simulink model "FOZN_BlueROV2_Control"  (R2023b)
settings: Solver=FixedStepAuto  StartTime=0.0  StopTime=600  FixedStep=0.01  RelTol=1e-3
values from neighbouring files (symbols this model uses):
  app_order = 5    [FOZN_controllers.m]
  Kp_heave = 0.2*Kc    (= 0.905736827128)    [RelayTest_controllerCalc.m]
  Kp_pitch = 0.2*Kc    (= 1.14706265291)    [RelayTest_controllerCalc.m]
  Kp_roll = 0.2*Kc    (= 0.102773850851)    [RelayTest_controllerCalc.m]
  Kp_surge = 0.2*Kc    (= 1.80686784967)    [RelayTest_controllerCalc.m]
  Kp_sway = 0.2*Kc    (= 0.383313460532)    [RelayTest_controllerCalc.m]
  Kp_yaw = 0.2*Kc    (= 0.127394021185)    [RelayTest_controllerCalc.m]
undefined symbols (not defined in the file or in its folder): Td_heave, Td_pitch, Td_roll, Td_surge, Td_sway, Td_yaw, Ti_heave, Ti_pitch, Ti_roll, Ti_surge, Ti_sway, Ti_yaw
libraries: fod x12
settings Model: Creator=tudor  LastModifiedBy=tudor

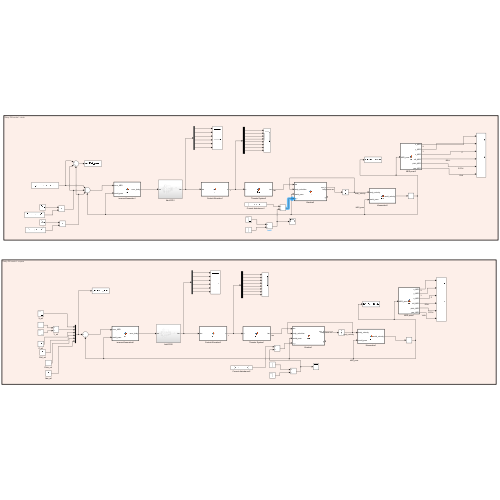
[thumbnail: Simulink's stored preview of the top-level diagram]
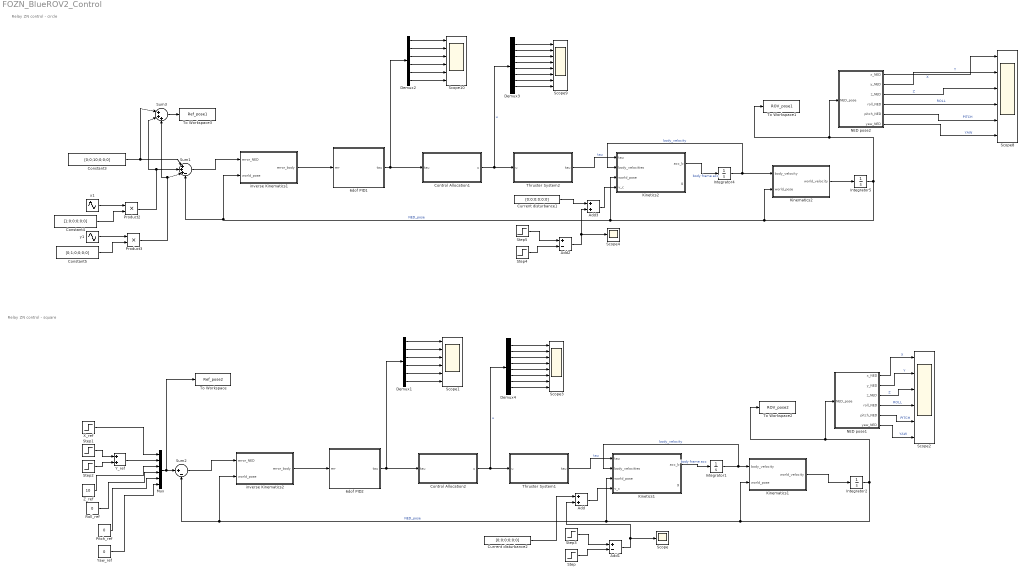
== system FOZN_BlueROV2_Control ==
  note: Relay ZN control - circle
  note: Relay ZN control - square
  6dof PID1 : Subsystem
  6dof PID2 : Subsystem
  Add : Sum
  Add1 : Sum  Inputs=+-
  Add2 : Sum  Inputs=+-
  Add3 : Sum
  Constant3 : Constant  Value=[0;0;10;0;0;0]
  Constant4 : Constant  Value=[1;0;0;0;0;0]
  Constant5 : Constant  Value=[0;1;0;0;0;0]
  Control Allocation1 : MATLAB Function  TreatAsAtomicUnit=on
  Control Allocation2 : MATLAB Function  TreatAsAtomicUnit=on
  Current disturbance1 : Constant  Value=[0;0;0;0;0;0]
  Current disturbance2 : Constant  Value=[0;0;0;0;0;0]
  Demux1 : Demux  Outputs=6
  Demux2 : Demux  Outputs=6
  Demux3 : Demux  Outputs=8
  Demux4 : Demux  Outputs=8
  Integrator1 : Integrator  InitialCondition=[0;0;0;0;0;0]
  Integrator2 : Integrator  InitialCondition=[0;0;10;0;0;0]
  Integrator4 : Integrator  InitialCondition=[0;0;0;0;0;0]
  Integrator5 : Integrator  InitialCondition=[0;0;10;0;0;0]
  Kinematics1 : MATLAB Function  TreatAsAtomicUnit=on
  Kinematics2 : MATLAB Function  TreatAsAtomicUnit=on
  Kinetics1 : MATLAB Function  TreatAsAtomicUnit=on
  Kinetics2 : MATLAB Function  TreatAsAtomicUnit=on
  Mux : Mux  Inputs=6
  NED pose1 : MATLAB Function  TreatAsAtomicUnit=on
  NED pose2 : MATLAB Function  TreatAsAtomicUnit=on
  Pitch_ref : Constant  Value=0
  Product2 : Product
  Product3 : Product
  Roll_ref : Constant  Value=0
  Scope : Scope
  Scope{1..2,8,10} (4 alike) : Scope  NumInputPorts=6
  Scope3 : Scope  NumInputPorts=8
  Scope4 : Scope
  Scope9 : Scope  NumInputPorts=8
  Step : Step  Time=100  Before=0.45  After=0  SampleTime=0
  Step1 : Step  Time=150  After=5  SampleTime=0
  Step2 : Step  Time=450  After=-5  SampleTime=0
  Step3 : Step  Time=125  Before=0.45  After=0  SampleTime=0
  Step4 : Step  Time=100  Before=0.45  After=0  SampleTime=0
  Step5 : Step  Time=125  Before=0.45  After=0  SampleTime=0
  Sum1 : Sum  Inputs=|+++-
  Sum2 : Sum  Inputs=|+-
  Sum3 : Sum  Inputs=|+++
  Thruster System1 : MATLAB Function  TreatAsAtomicUnit=on
  Thruster System2 : MATLAB Function  TreatAsAtomicUnit=on
  To Workspace : ToWorkspace  VariableName=Ref_pose2  SampleTime=-1
  To Workspace1 : ToWorkspace  VariableName=ROV_pose1  SampleTime=-1
  To Workspace2 : ToWorkspace  VariableName=ROV_pose2  SampleTime=-1
  To Workspace3 : ToWorkspace  VariableName=Ref_pose1  SampleTime=-1
  X_ref : Step  Time=300  Before=5  After=0  SampleTime=0
  Y_ref : Sum
  Yaw_ref : Constant  Value=0
  Z_ref : Constant  Value=10
  inverse Kinematics1 : MATLAB Function  TreatAsAtomicUnit=on
  inverse Kinematics2 : MATLAB Function  TreatAsAtomicUnit=on
  x1 : Sin  Frequency=0.1  SampleTime=0
  y1 : Sin  Frequency=0.1  Phase=pi/2  SampleTime=0
  wires:
  Demux2/6 -> Scope10/6
  Kinematics2/1(world_velocity) -> Integrator5/1
  Control Allocation1/1(u) -> Demux3/1, Thruster System2/1(u)  "u"
  NED pose2/6(yaw_NED) -> Scope8/6  "YAW"
  Demux3/3 -> Scope9/3
  Demux3/6 -> Scope9/6
  Demux3/2 -> Scope9/2
  Demux2/1 -> Scope10/1
  Kinetics2/1(acc_b) -> Integrator4/1  "body frame acc"
  Demux2/3 -> Scope10/3
  inverse Kinematics1/1(error_body) -> 6dof PID1/1(err)
  NED pose2/1(x_NED) -> Scope8/1  "X"
  Demux3/1 -> Scope9/1
  Current disturbance1/1 -> Add3/1
  Sum1/1 -> inverse Kinematics1/1(error_NED)
  Demux3/8 -> Scope9/8
  Integrator4/1 -> Kinetics2/2(body_velocities), Kinematics2/1(body_velocity)  "body_velocity"
  Demux3/7 -> Scope9/7
  Constant3/1 -> Sum3/1, Sum1/1
  6dof PID1/1(tau) -> Demux2/1, Control Allocation1/1(tau)
  Demux2/4 -> Scope10/4
  Thruster System2/1(tau) -> Kinetics2/1(tau)  "tau"
  Demux3/4 -> Scope9/4
  Integrator5/1 -> To Workspace1/1, NED pose2/1(NED_pose), Kinetics2/3(world_pose), Sum1/4, inverse Kinematics1/2(world_pose), Kinematics2/2(world_pose)  "NED_pose"
  NED pose2/2(y_NED) -> Scope8/2  "Y"
  NED pose2/4(roll_NED) -> Scope8/4  "ROLL"
  Demux2/2 -> Scope10/2
  NED pose2/3(z_NED) -> Scope8/3  "Z"
  Demux3/5 -> Scope9/5
  NED pose2/5(pitch_NED) -> Scope8/5  "PITCH"
  Demux2/5 -> Scope10/5
  Constant5/1 -> Product3/2
  Constant4/1 -> Product2/2
  y1/1 -> Product3/1
  Product2/1 -> Sum3/2, Sum1/2
  x1/1 -> Product2/1
  Product3/1 -> Sum1/3, Sum3/3
  X_ref/1 -> Mux/1
  Pitch_ref/1 -> Mux/5
  Step1/1 -> Y_ref/1
  Mux/1 -> To Workspace/1, Sum2/1
  Step2/1 -> Y_ref/2
  Y_ref/1 -> Mux/2
  Z_ref/1 -> Mux/3
  Yaw_ref/1 -> Mux/6
  Roll_ref/1 -> Mux/4
  6dof PID2/1(tau) -> Demux1/1, Control Allocation2/1(tau)
  Demux1/4 -> Scope1/4
  Demux4/8 -> Scope3/8
  Demux1/6 -> Scope1/6
  Control Allocation2/1(u) -> Demux4/1, Thruster System1/1(u)  "u"
  Kinematics1/1(world_velocity) -> Integrator2/1
  NED pose1/6(yaw_NED) -> Scope2/6  "YAW"
  Sum2/1 -> inverse Kinematics2/1(error_NED)
  Demux4/1 -> Scope3/1
  Demux1/1 -> Scope1/1
  Demux1/5 -> Scope1/5
  Kinetics1/1(acc_b) -> Integrator1/1  "body frame acc"
  NED pose1/4(roll_NED) -> Scope2/4  "ROLL"
  Thruster System1/1(tau) -> Kinetics1/1(tau)  "tau"
  Demux4/7 -> Scope3/7
  Demux1/3 -> Scope1/3
  Integrator2/1 -> To Workspace2/1, NED pose1/1(NED_pose), Kinetics1/3(world_pose), Sum2/2, inverse Kinematics2/2(world_pose), Kinematics1/2(world_pose)  "NED_pose"
  NED pose1/1(x_NED) -> Scope2/1  "X"
  inverse Kinematics2/1(error_body) -> 6dof PID2/1(err)
  Demux4/4 -> Scope3/4
  Demux4/6 -> Scope3/6
  Current disturbance2/1 -> Add/1
  NED pose1/5(pitch_NED) -> Scope2/5  "PITCH"
  Demux4/3 -> Scope3/3
  NED pose1/2(y_NED) -> Scope2/2  "Y"
  Demux4/2 -> Scope3/2
  Demux1/2 -> Scope1/2
  Integrator1/1 -> Kinetics1/2(body_velocities), Kinematics1/1(body_velocity)  "body_velocity"
  Demux4/5 -> Scope3/5
  NED pose1/3(z_NED) -> Scope2/3  "Z"
  Add/1 -> Kinetics1/4(v_c)
  Step3/1 -> Add1/1
  Step/1 -> Add1/2
  Add1/1 -> Scope/1, Add/2
  Sum3/1 -> To Workspace3/1
  Add2/1 -> Add3/2, Scope4/1
  Step4/1 -> Add2/2
  Step5/1 -> Add2/1
  Add3/1 -> Kinetics2/4(v_c)

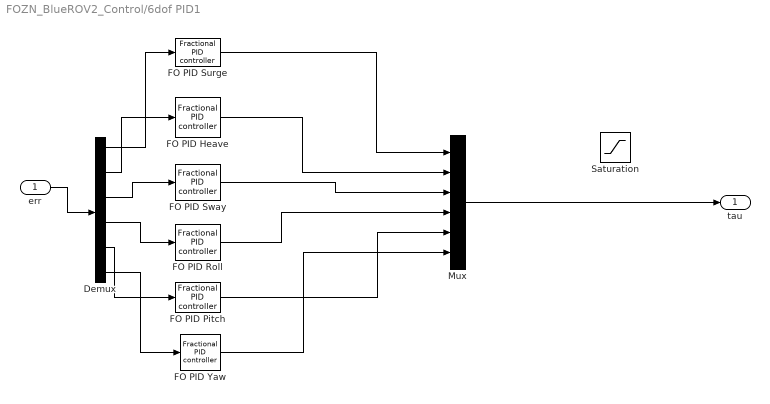
== system FOZN_BlueROV2_Control/6dof PID1 ==
  err : Inport
  Demux : Demux  Outputs=6
  FO PID Heave : fod/Fractional PID controller  Kp=Kp_heave  Ki=Kp_heave/Ti_heave  lambda=lambda_heave  Kd=Kp_heave*Td_heave  mic=lambda_heave  freqRange=freq_range  N=app_order
      settings: SourceProductName=FOMCON Toolbox
  FO PID Pitch : fod/Fractional PID controller  Kp=Kp_pitch  Ki=Kp_pitch/Ti_pitch  lambda=lambda_pitch  Kd=Kp_pitch*Td_pitch  mic=lambda_pitch  freqRange=freq_range  N=app_order
      settings: SourceProductName=FOMCON Toolbox
  FO PID Roll : fod/Fractional PID controller  Kp=Kp_roll  Ki=Kp_roll/Ti_roll  lambda=lambda_roll  Kd=Kp_roll*Td_roll  mic=lambda_roll  freqRange=freq_range  N=app_order
      settings: SourceProductName=FOMCON Toolbox
  FO PID Surge : fod/Fractional PID controller  Kp=Kp_surge  Ki=Kp_surge/Ti_surge  lambda=lambda_surge  Kd=Kp_surge*Td_surge  mic=lambda_surge  freqRange=freq_range  N=app_order
      settings: SourceProductName=FOMCON Toolbox
  FO PID Sway : fod/Fractional PID controller  Kp=Kp_sway  Ki=Kp_sway/Ti_sway  lambda=lambda_sway  Kd=Kp_sway*Td_sway  mic=lambda_sway  freqRange=freq_range  N=app_order
      settings: SourceProductName=FOMCON Toolbox
  FO PID Yaw : fod/Fractional PID controller  Kp=Kp_yaw  Ki=Kp_yaw/Ti_yaw  lambda=lambda_yaw  Kd=Kp_yaw*Td_yaw  mic=lambda_yaw  freqRange=freq_range  N=app_order
      settings: SourceProductName=FOMCON Toolbox
  Mux : Mux  Inputs=6
  Saturation : Saturate  UpperLimit=16  LowerLimit=-16
  tau : Outport
  wires:
  Demux/6 -> FO PID Yaw/1
  err/1 -> Demux/1
  Mux/1 -> tau/1
  Demux/1 -> FO PID Surge/1
  Demux/3 -> FO PID Sway/1
  Demux/2 -> FO PID Heave/1
  Demux/4 -> FO PID Roll/1
  Demux/5 -> FO PID Pitch/1
  FO PID Yaw/1 -> Mux/6
  FO PID Surge/1 -> Mux/1
  FO PID Heave/1 -> Mux/2
  FO PID Sway/1 -> Mux/3
  FO PID Roll/1 -> Mux/4
  FO PID Pitch/1 -> Mux/5

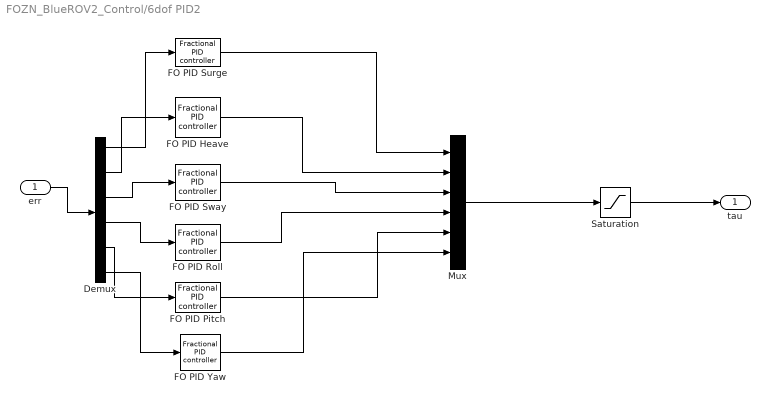
== system FOZN_BlueROV2_Control/6dof PID2 ==
  err : Inport
  Demux : Demux  Outputs=6
  FO PID Heave : fod/Fractional PID controller  Kp=Kp_heave  Ki=Kp_heave/Ti_heave  lambda=lambda_heave  Kd=Kp_heave*Td_heave  mic=lambda_heave  freqRange=freq_range  N=app_order
      settings: SourceProductName=FOMCON Toolbox
  FO PID Pitch : fod/Fractional PID controller  Kp=Kp_pitch  Ki=Kp_pitch/Ti_pitch  lambda=lambda_pitch  Kd=Kp_pitch*Td_pitch  mic=lambda_pitch  freqRange=freq_range  N=app_order
      settings: SourceProductName=FOMCON Toolbox
  FO PID Roll : fod/Fractional PID controller  Kp=Kp_roll  Ki=Kp_roll/Ti_roll  lambda=lambda_roll  Kd=Kp_roll*Td_roll  mic=lambda_roll  freqRange=freq_range  N=app_order
      settings: SourceProductName=FOMCON Toolbox
  FO PID Surge : fod/Fractional PID controller  Kp=Kp_surge  Ki=Kp_surge/Ti_surge  lambda=lambda_surge  Kd=Kp_surge*Td_surge  mic=lambda_surge  freqRange=freq_range  N=app_order
      settings: SourceProductName=FOMCON Toolbox
  FO PID Sway : fod/Fractional PID controller  Kp=Kp_sway  Ki=Kp_sway/Ti_sway  lambda=lambda_sway  Kd=Kp_sway*Td_sway  mic=lambda_sway  freqRange=freq_range  N=app_order
      settings: SourceProductName=FOMCON Toolbox
  FO PID Yaw : fod/Fractional PID controller  Kp=Kp_yaw  Ki=Kp_yaw/Ti_yaw  lambda=lambda_yaw  Kd=Kp_yaw*Td_yaw  mic=lambda_yaw  freqRange=freq_range  N=app_order
      settings: SourceProductName=FOMCON Toolbox
  Mux : Mux  Inputs=6
  Saturation : Saturate  UpperLimit=500  LowerLimit=-500
  tau : Outport
  wires:
  Demux/6 -> FO PID Yaw/1
  err/1 -> Demux/1
  Mux/1 -> Saturation/1
  Demux/1 -> FO PID Surge/1
  Demux/3 -> FO PID Sway/1
  Demux/2 -> FO PID Heave/1
  Demux/4 -> FO PID Roll/1
  Demux/5 -> FO PID Pitch/1
  FO PID Yaw/1 -> Mux/6
  FO PID Surge/1 -> Mux/1
  FO PID Heave/1 -> Mux/2
  FO PID Sway/1 -> Mux/3
  FO PID Roll/1 -> Mux/4
  FO PID Pitch/1 -> Mux/5
  Saturation/1 -> tau/1

== matlab function FOZN_BlueROV2_Control/Thruster System2 ==
  data: u input; tau output
function tau = fcn(u)
%The BlueROV2 heavy has an 8 thruster configuration: u is R^8.
%This function maps the PWM control input into generalised forces and
%moments of a 6 DoF with a specific 8 thruster configuration.


%Assuming linearity, the control force due to a thruster can be represented
%as F=Ku, with K is R^(8x8), diagonal. Using the BlueROV2 datasheed, the
%thrust coefficient matrix K is:
K=40*eye(8);

%We have to take into account the thrust configuration matrix (angle of
%each thruster with respect to the local XYZ (NED) frame attached 
%to the ROV:
T=[0.707    0.707   -0.707  -0.707      0       0     0     0;
   -0.707   0.707   -0.707   0.707      0       0     0     0;
      0        0        0       0      -1       1     1    -1;
    0.06    -0.06     0.06   -0.06  -0.218 -0.218 0.218  0.218;
    0.06     0.06    -0.06   -0.06   0.120 -0.120 0.120 -0.120;
  -0.1888  0.1888   0.1888  -0.1888    0      0     0      0];


tau = T*K*u;

== matlab function FOZN_BlueROV2_Control/inverse Kinematics1 ==
  data: error_NED input; error_body output; world_pose input
function error_body = fcn(error_NED,world_pose)

psi=world_pose(6);
theta=world_pose(5);
phi=world_pose(4);
%Getting the linear and angular velocites from body frame to NED world
%frame. The used orientation convention is Euler Angles -> Roll Pitch Yaw.
Rz=[cos(psi)  -sin(psi)  0;
    sin(psi)   cos(psi)  0;
       0           0     1];

Ry=[cos(theta)   0     sin(theta);
       0         1        0;
    -sin(theta)  0    cos(theta)];

Rx=[1      0          0;
    0   cos(phi)  -sin(phi);
    0   sin(phi)   cos(phi)];

R_bn=Rz*Ry*Rx;

T=[1 sin(phi)*tan(theta) cos(phi)*tan(theta);
   0        cos(phi)            -sin(phi);
   0 sin(phi)/cos(theta) cos(phi)*cos(theta)];

J=[R_bn         zeros([3,3]);
  zeros([3,3])          T];

 error_body= inv(J)*error_NED;

== matlab function FOZN_BlueROV2_Control/Control Allocation2 ==
  data: tau input; u output
function u = fcn(tau)
%The BlueROV2 heavy has an 8 thruster configuration: u is R^8.
%This function maps the PWM control input into generalised forces and
%moments of a 6 DoF with a specific 8 thruster configuration.


%Assuming linearity, the control force due to a thruster can be represented
%as F=Ku, with K is R^(8x8), diagonal. Using the BlueROV2 datasheed, the
%thrust coefficient matrix K is:
K=40*eye(8);

%We have to take into account the thrust configuration matrix (angle of
%each thruster with respect to the local XYZ (NED) frame attached 
%to the ROV:
T=[0.707    0.707   -0.707  -0.707      0       0     0     0;
   -0.707   0.707   -0.707   0.707      0       0     0     0;
      0        0        0       0      -1       1     1    -1;
    0.06    -0.06     0.06   -0.06  -0.218 -0.218 0.218  0.218;
    0.06     0.06    -0.06   -0.06   0.120 -0.120 0.120 -0.120;
  -0.1888  0.1888   0.1888  -0.1888    0      0     0      0];


u = inv(K)*pinv(T)*tau;

== matlab function FOZN_BlueROV2_Control/Kinematics1 ==
  data: body_velocity input; world_velocity output; world_pose input
function world_velocity = fcn(body_velocity,world_pose)

psi=world_pose(6);
theta=world_pose(5);
phi=world_pose(4);
%Getting the linear and angular velocites from body frame to NED world
%frame. The used orientation convention is Euler Angles -> Roll Pitch Yaw.
Rz=[cos(psi)  -sin(psi)  0;
    sin(psi)   cos(psi)  0;
       0           0     1];

Ry=[cos(theta)   0     sin(theta);
       0         1        0;
    -sin(theta)  0    cos(theta)];

Rx=[1      0          0;
    0   cos(phi)  -sin(phi);
    0   sin(phi)   cos(phi)];

R_bn=Rz*Ry*Rx;

T=[1 sin(phi)*tan(theta) cos(phi)*tan(theta);
   0        cos(phi)            -sin(phi);
   0 sin(phi)/cos(theta) cos(phi)*cos(theta)];

J=[R_bn         zeros([3,3]);
  zeros([3,3])          T];

world_velocity = J*body_velocity;

== matlab function FOZN_BlueROV2_Control/Kinetics1 ==
  data: tau input; body_velocities input; world_pose input; acc_b output; v_c input; g output
function [acc_b, g] = fcn(tau,body_velocities,world_pose,v_c)
%The acceleration in body frame is determined 
%using the kinetic dynamic equations (Newton Euler):
%M_RB*dv + C_RB*v + M_A*dv_w + C_A*v_w + D*v_w + g = tau, where
%vw=v-v_c, where v_c is the speed of the waves - disturbances.

phi=world_pose(4);
theta=world_pose(5);
psi=world_pose(6);


u=body_velocities(1);
v=body_velocities(2);
w=body_velocities(3);
p=body_velocities(4);
q=body_velocities(5);
r=body_velocities(6);

%We shall first define some constants:
%ROV mass:
m=11.5;
%ROV weight
W=112.8;
%Buoyancy force
B=114.8;
%we place the centre of buoyancy in the center of the body frame:
rb=[0;0;0];
%position of the center of gravity w.r.t. the centre of buoyancy:
rg=[0;0;0.02];%in reality is 0.00019
%inertia moments about x,y,z in body frame are:
Ix=0.16; Iy=0.16; Iz=0.16;

%Added mass parameters:
X_du=-5.5; Y_dv=-12.7; Z_dw=-14.57; K_dp=-0.12; M_dq=-0.12; N_dr=-0.12;

%linear (e.g.X_u) and quadratic (e.g.X_u2 ->X_u|u|) dampig parameters:
X_u=-4.03; Y_v=-6.22; Z_w=-5.18; K_p=-0.07; M_q=-0.07; N_r=-0.07;
X_u2=-18.18; Y_v2=-21.66; Z_w2=-36.99; K_p2=-1.55; M_q2=-1.55; N_r2=-1.55;


M_RB =[m        0       0       0       m*rb(3)      0;
       0        m       0     -m*rb(3)    0          0;
       0        0       m       0         0          0;
       0      -m*rb(3)  0       Ix        0          0;
       m*rb(3)  0       0       0         Iy         0;
       0        0       0       0         0          Iz];
%u,v,w are linear velocities and p,q,r are angular velocities represented
%in body frame
C_RB =[0     0    0    0      m*w     0;
       0     0    0  -m*w      0      0;
       0     0    0   m*v    -m*u     0;
       0    m*w -m*v   0     Iz*r  -Iy*q;
     -m*w    0  -m*u -Iz*r     0    Ix*p;
      m*v  -m*u   0   Iy*q  -Ix*p     0]; 

% M_A = diag([X_du Y_dv Z_dw K_dp M_dq N_dr]);
% 
% C_A =[0     0       0       0     Z_dw*w       0;
%       0     0       0    -Z_dw*w     0       -X_du*u;
%       0     0       0    -Y_dv*v  X_du*u       0;
%       0   -Z_dw*w  Y_dv*v  0      -N_dr*r     M_dq*q;
%     Z_dw*w  0     -X_du*u N_dr*r    0        -K_dp*p;
%    -Y_dv*v X_du*u   0    -M_dq*q   K_dp*p      0];

%The Hydrodynamic damping can be approx with a linear damping D_L and a
%quadratic damping D_NL
D_L=-diag([X_u Y_v Z_w K_p M_q N_r]);

D_NL=-diag([X_u2*abs(u) Y_v2*abs(v) Z_w2*abs(w)...
           K_p2*abs(p) M_q2*abs(q) N_r2*abs(r)]);

D = D_L + D_NL;

%gravitational and
g = [(W-B)*sin(theta);
     -(W-B)*cos(theta)*sin(phi);
     -(W-B)*cos(theta)*cos(phi);
     rb(3)*W*cos(theta)*sin(phi);
     rb(3)*W*sin(theta);
     0];

%g = 0;

%with Ma and Ca
% acc_b=inv(M_RB+M_A)*(tau-C_RB*body_velocities ...
%                     -C_A*(body_velocities-v_c)-D*(body_velocities-v_c)-g);


%without Ma and Ca
acc_b=inv(M_RB)*(tau-C_RB*body_velocities-D*(body_velocities-v_c)-g);

== matlab function FOZN_BlueROV2_Control/NED pose1 ==
  data: NED_pose input; x_NED output; y_NED output; z_NED output; roll_NED output; pitch_NED output; yaw_NED output
function [x_NED,y_NED,z_NED,roll_NED,pitch_NED,yaw_NED] = fcn(NED_pose)

x_NED =NED_pose(1);
y_NED =NED_pose(2);
z_NED =NED_pose(3);
roll_NED=NED_pose(4);
pitch_NED =NED_pose(5);
yaw_NED=NED_pose(6);

== matlab function FOZN_BlueROV2_Control/Thruster System1 ==
  data: u input; tau output
function tau = fcn(u)
%The BlueROV2 heavy has an 8 thruster configuration: u is R^8.
%This function maps the PWM control input into generalised forces and
%moments of a 6 DoF with a specific 8 thruster configuration.


%Assuming linearity, the control force due to a thruster can be represented
%as F=Ku, with K is R^(8x8), diagonal. Using the BlueROV2 datasheed, the
%thrust coefficient matrix K is:
K=40*eye(8);

%We have to take into account the thrust configuration matrix (angle of
%each thruster with respect to the local XYZ (NED) frame attached 
%to the ROV:
T=[0.707    0.707   -0.707  -0.707      0       0     0     0;
   -0.707   0.707   -0.707   0.707      0       0     0     0;
      0        0        0       0      -1       1     1    -1;
    0.06    -0.06     0.06   -0.06  -0.218 -0.218 0.218  0.218;
    0.06     0.06    -0.06   -0.06   0.120 -0.120 0.120 -0.120;
  -0.1888  0.1888   0.1888  -0.1888    0      0     0      0];


tau = T*K*u;

== matlab function FOZN_BlueROV2_Control/inverse Kinematics2 ==
  data: error_NED input; error_body output; world_pose input
function error_body = fcn(error_NED,world_pose)

psi=world_pose(6);
theta=world_pose(5);
phi=world_pose(4);
%Getting the linear and angular velocites from body frame to NED world
%frame. The used orientation convention is Euler Angles -> Roll Pitch Yaw.
Rz=[cos(psi)  -sin(psi)  0;
    sin(psi)   cos(psi)  0;
       0           0     1];

Ry=[cos(theta)   0     sin(theta);
       0         1        0;
    -sin(theta)  0    cos(theta)];

Rx=[1      0          0;
    0   cos(phi)  -sin(phi);
    0   sin(phi)   cos(phi)];

R_bn=Rz*Ry*Rx;

T=[1 sin(phi)*tan(theta) cos(phi)*tan(theta);
   0        cos(phi)            -sin(phi);
   0 sin(phi)/cos(theta) cos(phi)*cos(theta)];

J=[R_bn         zeros([3,3]);
  zeros([3,3])          T];

 error_body= inv(J)*error_NED;

== matlab function FOZN_BlueROV2_Control/Control Allocation1 ==
  data: tau input; u output
function u = fcn(tau)
%The BlueROV2 heavy has an 8 thruster configuration: u is R^8.
%This function maps the PWM control input into generalised forces and
%moments of a 6 DoF with a specific 8 thruster configuration.


%Assuming linearity, the control force due to a thruster can be represented
%as F=Ku, with K is R^(8x8), diagonal. Using the BlueROV2 datasheed, the
%thrust coefficient matrix K is:
K=40*eye(8);

%We have to take into account the thrust configuration matrix (angle of
%each thruster with respect to the local XYZ (NED) frame attached 
%to the ROV:
T=[0.707    0.707   -0.707  -0.707      0       0     0     0;
   -0.707   0.707   -0.707   0.707      0       0     0     0;
      0        0        0       0      -1       1     1    -1;
    0.06    -0.06     0.06   -0.06  -0.218 -0.218 0.218  0.218;
    0.06     0.06    -0.06   -0.06   0.120 -0.120 0.120 -0.120;
  -0.1888  0.1888   0.1888  -0.1888    0      0     0      0];


u = inv(K)*pinv(T)*tau;

== matlab function FOZN_BlueROV2_Control/Kinematics2 ==
  data: body_velocity input; world_velocity output; world_pose input
function world_velocity = fcn(body_velocity,world_pose)

psi=world_pose(6);
theta=world_pose(5);
phi=world_pose(4);
%Getting the linear and angular velocites from body frame to NED world
%frame. The used orientation convention is Euler Angles -> Roll Pitch Yaw.
Rz=[cos(psi)  -sin(psi)  0;
    sin(psi)   cos(psi)  0;
       0           0     1];

Ry=[cos(theta)   0     sin(theta);
       0         1        0;
    -sin(theta)  0    cos(theta)];

Rx=[1      0          0;
    0   cos(phi)  -sin(phi);
    0   sin(phi)   cos(phi)];

R_bn=Rz*Ry*Rx;

T=[1 sin(phi)*tan(theta) cos(phi)*tan(theta);
   0        cos(phi)            -sin(phi);
   0 sin(phi)/cos(theta) cos(phi)*cos(theta)];

J=[R_bn         zeros([3,3]);
  zeros([3,3])          T];

world_velocity = J*body_velocity;

== matlab function FOZN_BlueROV2_Control/Kinetics2 ==
  data: tau input; body_velocities input; world_pose input; acc_b output; v_c input; g output
function [acc_b, g] = fcn(tau,body_velocities,world_pose,v_c)
%The acceleration in body frame is determined 
%using the kinetic dynamic equations (Newton Euler):
%M_RB*dv + C_RB*v + M_A*dv_w + C_A*v_w + D*v_w + g = tau, where
%vw=v-v_c, where v_c is the speed of the waves - disturbances.

phi=world_pose(4);
theta=world_pose(5);
psi=world_pose(6);


u=body_velocities(1);
v=body_velocities(2);
w=body_velocities(3);
p=body_velocities(4);
q=body_velocities(5);
r=body_velocities(6);

%We shall first define some constants:
%ROV mass:
m=11.5;
%ROV weight
W=112.8;
%Buoyancy force
B=114.8;
%we place the centre of buoyancy in the center of the body frame:
rb=[0;0;0];
%position of the center of gravity w.r.t. the centre of buoyancy:
rg=[0;0;0.02];%in reality is 0.00019
%inertia moments about x,y,z in body frame are:
Ix=0.16; Iy=0.16; Iz=0.16;

%Added mass parameters:
X_du=-5.5; Y_dv=-12.7; Z_dw=-14.57; K_dp=-0.12; M_dq=-0.12; N_dr=-0.12;

%linear (e.g.X_u) and quadratic (e.g.X_u2 ->X_u|u|) dampig parameters:
X_u=-4.03; Y_v=-6.22; Z_w=-5.18; K_p=-0.07; M_q=-0.07; N_r=-0.07;
X_u2=-18.18; Y_v2=-21.66; Z_w2=-36.99; K_p2=-1.55; M_q2=-1.55; N_r2=-1.55;


M_RB =[m        0       0       0       m*rb(3)      0;
       0        m       0     -m*rb(3)    0          0;
       0        0       m       0         0          0;
       0      -m*rb(3)  0       Ix        0          0;
       m*rb(3)  0       0       0         Iy         0;
       0        0       0       0         0          Iz];
%u,v,w are linear velocities and p,q,r are angular velocities represented
%in body frame
C_RB =[0     0    0    0      m*w     0;
       0     0    0  -m*w      0      0;
       0     0    0   m*v    -m*u     0;
       0    m*w -m*v   0     Iz*r  -Iy*q;
     -m*w    0  -m*u -Iz*r     0    Ix*p;
      m*v  -m*u   0   Iy*q  -Ix*p     0]; 

% M_A = diag([X_du Y_dv Z_dw K_dp M_dq N_dr]);
% 
% C_A =[0     0       0       0     Z_dw*w       0;
%       0     0       0    -Z_dw*w     0       -X_du*u;
%       0     0       0    -Y_dv*v  X_du*u       0;
%       0   -Z_dw*w  Y_dv*v  0      -N_dr*r     M_dq*q;
%     Z_dw*w  0     -X_du*u N_dr*r    0        -K_dp*p;
%    -Y_dv*v X_du*u   0    -M_dq*q   K_dp*p      0];

%The Hydrodynamic damping can be approx with a linear damping D_L and a
%quadratic damping D_NL
D_L=-diag([X_u Y_v Z_w K_p M_q N_r]);

D_NL=-diag([X_u2*abs(u) Y_v2*abs(v) Z_w2*abs(w)...
           K_p2*abs(p) M_q2*abs(q) N_r2*abs(r)]);

D = D_L + D_NL;

%gravitational and
g = [(W-B)*sin(theta);
     -(W-B)*cos(theta)*sin(phi);
     -(W-B)*cos(theta)*cos(phi);
     rb(3)*W*cos(theta)*sin(phi);
     rb(3)*W*sin(theta);
     0];

%g = 0;

%with Ma and Ca
% acc_b=inv(M_RB+M_A)*(tau-C_RB*body_velocities ...
%                     -C_A*(body_velocities-v_c)-D*(body_velocities-v_c)-g);


%without Ma and Ca
acc_b=inv(M_RB)*(tau-C_RB*body_velocities-D*(body_velocities-v_c)-g);

== matlab function FOZN_BlueROV2_Control/NED pose2 ==
  data: NED_pose input; x_NED output; y_NED output; z_NED output; roll_NED output; pitch_NED output; yaw_NED output
function [x_NED,y_NED,z_NED,roll_NED,pitch_NED,yaw_NED] = fcn(NED_pose)

x_NED =NED_pose(1);
y_NED =NED_pose(2);
z_NED =NED_pose(3);
roll_NED=NED_pose(4);
pitch_NED =NED_pose(5);
yaw_NED=NED_pose(6);
